simulink model "WEankle_controllerMaarten_TimingPerturb_2018"  (R2018a)
settings: Solver=FixedStepDiscrete  StartTime=0.0  StopTime=inf  FixedStep=sampleTime  RelTol=1e-3
undefined symbols (not defined in the file or in its folder): DiscIntNeverNeededParam, forceplate
libraries: simulink x17, WE2_library x8, dspsigops x6, dspfdesign x3
(part 3 of 3)

== matlab function WEankle_controllerMaarten_TimingPerturb_2018/Ankle Controller/AnkleControllerGeyer/Muscle Geometry ==
  data: q input; lMT output; dM output; qOffsetLeft input; qOffsetRight input
function [lMT,dM] = GetMuscleGeometry_Simulink(q,qOffsetLeft,qOffsetRight)
% GetMuscleGeometry is a function that uses polynomials to evaluate the muscle-tendon
% lengths, velocities and  moment arms as a function of the joint angles and velocities.
% Inputs:
%   - q: vector with joint angles
% Outputs:
%   - lMT: muscle-tendon length
%   - dM: moment arm

lMT = zeros(4,1);
dM = zeros(4,1);

qrel = q - [qOffsetLeft; qOffsetRight];

for i = 1:length(qrel)
    if  qrel(i) < -15*pi/180
        qrel(i) = -15*pi/180;
    end
    if  qrel(i) > 15*pi/180
        qrel(i) = 15*pi/180;
    end
end

% use matlab function to get muscle geometry
[lMT_Left,dM_Left] = GetMuscleGeometry_LengthOnly(-qrel(1));
[lMT_Right,dM_Right] = GetMuscleGeometry_LengthOnly(-qrel(2));

lMT = [lMT_Left; lMT_Right];
dM = [dM_Left; dM_Right];

end

== matlab function WEankle_controllerMaarten_TimingPerturb_2018/Ankle Controller/AnkleControllerGeyer/MATLAB Function1 ==
  data: GRFy_Left input; GRFy_Right input; e output; Ftilde input; lMtilde input; COMd input; SoleusGains input; TibialisGains input; BodyMass input
function e  = GeyerAnkleModel_Simulink(GRFy_Left,GRFy_Right,Ftilde,lMtilde, COMd, SoleusGains, TibialisGains, BodyMass )
% input arguments:

% extract structure with gains from gains vector (makes it easier to read)
Gains = ExtractGains(SoleusGains,TibialisGains);

% compute excitations based on feedback models
[eLeft] = GeyerAnkle(GRFy_Left,Gains,Ftilde(1),lMtilde(2),COMd, BodyMass);
[eRight] = GeyerAnkle(GRFy_Right,Gains,Ftilde(3),lMtilde(4),COMd, BodyMass);

% vector with excitations
e =[eLeft; eRight];

== matlab function WEankle_controllerMaarten_TimingPerturb_2018/Ankle Controller/AnkleControllerGeyer/ActivationDynamics1 ==
  data: e input; dadt output; a input
function dadt = ActDyn(e,a)

% See publication (DeGroote2016), equations 1-2, for more details
% (note tanh implementation mainly needed for gradient based optimization.
% Not needed in the actual controller. (I decided to keep it so that the
% dynamics of the parameter estimation and the controller are exactly the
% same

% tact = 0.02;
% tdeact = 0.04;

% contraction dynamics with smooth transition
% b = 0.001;
% d1 = 1./(tact.*(0.5+1.5*a));
% d2 = (0.5+1.5*a)./tdeact;
% f = 0.5*tanh(b*(e-a));
% dadt = (d1.*(f+0.5) + d2.*(-f+0.5)).*(e-a);

% try explicit version of contraction dynamics ( error in twincat with
% smooth version
% dadt = zeros(4,1);
% for i=1:length(a)
%     if a(i) < e(i)
%         tau_sel = tact;
%     else
%         tau_sel = tdeact;
%     end
%     dadt(i) = (e(i)-a(i))./ tau_sel;    
% end

% dadt = zeros(4,1);
% for i=1:length(a)   
%     dadt(i) = (e(i)-a(i))./ 0.03;    
% end

dadt = (e-a)./0.03;

== matlab function WEankle_controllerMaarten_TimingPerturb_2018/Ankle Controller/AnkleControllerGeyer/ContractionDynamics1 ==
  data: a input; dlMdt output; lMtilde input; lMT input; F output; Fce_tilde output
function [dlMdt, F , Fce_tilde] = ContractionDynamics_Simulink(a,lMtilde,lMT)
% ContractionDynamics_Simulink Simulates contraction dynamics

% Muscle contraction dynamics left leg
[dlMdt_Left, F_Left , Fce_tilde_Left] = MuscleContractionDynamics(a(1:2),lMtilde(1:2),lMT(1:2));
 
% Muscle contraction dynamics right leg
[dlMdt_Right, F_Right , Fce_tilde_Right] = MuscleContractionDynamics(a(3:4),lMtilde(3:4),lMT(3:4));

% combine vectors
dlMdt = [dlMdt_Left; dlMdt_Right];
F = [F_Left; F_Right];
Fce_tilde = [Fce_tilde_Left; Fce_tilde_Right];

== matlab function WEankle_controllerMaarten_TimingPerturb_2018/Ankle Controller/AnkleControllerGeyer/ComputeJointMoment ==
  data: F input; tauModel output; dM input
function tauModel  = ComputeJointMoment(F,dM)

% matlab function to compute muscle contraction dynamics
tauLeft = dM(1).*F(1) + dM(2).*F(2);
tauRight = dM(3).*F(3) + dM(4).*F(4);
tauModel = [tauLeft; tauRight];

== matlab function WEankle_controllerMaarten_TimingPerturb_2018/Ankle Controller/AnkleControllerGeyer1/ContractionDynamics2 ==
  data: F input; tauModel output; dM input
function tauModel  = ComputeJointMoment(F,dM)

% matlab function to compute muscle contraction dynamics
tauLeft = dM(1).*F(1) + dM(2).*F(2);
tauRight = dM(3).*F(3) + dM(4).*F(4);
tauModel = [tauLeft; tauRight];

== matlab function WEankle_controllerMaarten_TimingPerturb_2018/Ankle Controller/AnkleControllerGeyer1/MATLAB Function1 ==
  data: GRFy_Left input; GRFy_Right input; e output; Ftilde input; lMtilde input; COMd input; SoleusGains input; TibialisGains input; BodyMass input
function e  = GeyerAnkleModel_Simulink(GRFy_Left,GRFy_Right,Ftilde,lMtilde, COMd, SoleusGains, TibialisGains, BodyMass )
% input arguments:

% extract structure with gains from gains vector (makes it easier to read)
Gains = ExtractGains(SoleusGains,TibialisGains);

% compute excitations based on feedback models
[eLeft] = GeyerAnkle(GRFy_Left,Gains,Ftilde(1),lMtilde(2),COMd, BodyMass);
[eRight] = GeyerAnkle(GRFy_Right,Gains,Ftilde(3),lMtilde(4),COMd, BodyMass);

% vector with excitations
e =[eLeft; eRight];

== matlab function WEankle_controllerMaarten_TimingPerturb_2018/Ankle Controller/AnkleControllerGeyer1/Muscle Geometry ==
  data: q input; lMT output; dM output; qOffsetLeft input; qOffsetRight input
function [lMT,dM] = GetMuscleGeometry_Simulink(q,qOffsetLeft,qOffsetRight)
% GetMuscleGeometry is a function that uses polynomials to evaluate the muscle-tendon
% lengths, velocities and  moment arms as a function of the joint angles and velocities.
% Inputs:
%   - q: vector with joint angles
% Outputs:
%   - lMT: muscle-tendon length
%   - dM: moment arm

lMT = zeros(4,1);
dM = zeros(4,1);

qrel = q - [qOffsetLeft; qOffsetRight];

for i = 1:length(qrel)
    if  qrel(i) < -15*pi/180
        qrel(i) = -15*pi/180;
    end
    if  qrel(i) > 15*pi/180
        qrel(i) = 15*pi/180;
    end
end

% use matlab function to get muscle geometry
[lMT_Left,dM_Left] = GetMuscleGeometry_LengthOnly(-qrel(1));
[lMT_Right,dM_Right] = GetMuscleGeometry_LengthOnly(-qrel(2));

lMT = [lMT_Left; lMT_Right];
dM = [dM_Left; dM_Right];

end

== matlab function WEankle_controllerMaarten_TimingPerturb_2018/Ankle Controller/MATLAB Function9 ==
  data: tau_Reflex input; tau_ReflexUnp input; tau_Left output; BodyMass input; BodyLength input; tau_Right output; MaxTorque input; TorqueScale input; ControlType input
function [tau_Left, tau_Right]  = DesiredExoMoment(tau_Reflex, tau_ReflexUnp,...
    BodyMass, BodyLength, MaxTorque, TorqueScale,ControlType)
%DesiredExoMoment switched between control types and selects the desired
%exo moment for the left and right leg

[tau_Left, tau_Right]  = f_DesiredExoMoment(tau_Reflex, tau_ReflexUnp,...
    BodyMass, BodyLength, MaxTorque, TorqueScale,ControlType);

== matlab function WEankle_controllerMaarten_TimingPerturb_2018/GetAnkleAngleStanding/MATLAB Function ==
  data: q input; qLeft output; start input; caltime_s input; qRight output
function [qLeft, qRight] = EncoderOffset_GeyerModel(q, start, caltime_s)
% q = joint angle
% start = boolean indicate start callibration is triggered
% caltime_s = total callibration time

qLeft = f_EncoderOffset_GeyerModel(q(1),start,caltime_s);
qRight = f_EncoderOffset_GeyerModel(q(2),start,caltime_s);
